simulink model "ex8_1"  (R2020a)
settings: Solver=ode45  StartTime=-pi/4  StopTime=pi/4  RelTol=1e-3
libraries: simulink x1
settings Model: Creator=반달  LastModifiedBy=반달
settings DataIOCC: ReturnWorkspaceOutputs=off

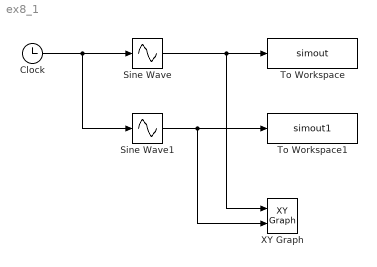
== system ex8_1 ==
  Clock : Clock
  Sine Wave : Sin  TimeSource=Use external signal  Amplitude=0.8  Phase=pi/2  SampleTime=0
  Sine Wave1 : Sin  TimeSource=Use external signal  Amplitude=0.8  SampleTime=0
  To Workspace : ToWorkspace  VariableName=simout  SaveFormat=Structure With Time  SampleTime=-1
  To Workspace1 : ToWorkspace  VariableName=simout1  SaveFormat=Structure With Time  SampleTime=-1
  XY Graph : simulink/Sinks/XY Graph  xmin=-1  xmax=1  ymin=-1  ymax=1  st=-1
  wires:
  Sine Wave1/1 -> To Workspace1/1, XY Graph/2
  Sine Wave/1 -> To Workspace/1, XY Graph/1
  Clock/1 -> Sine Wave/1, Sine Wave1/1
